simulink model "rocket_thrust_data_test"  (R2014a)
settings: Solver=ode45  StartTime=0.0  StopTime=1.3  MinStep=0.01  RelTol=1e-3
libraries: rocket_thrust_data_library x1, rocket_dynamic_data_library x1
settings Model: Creator=scorpii  LastModifiedBy=scorpii
settings SolverCC: InitialStep=0.01

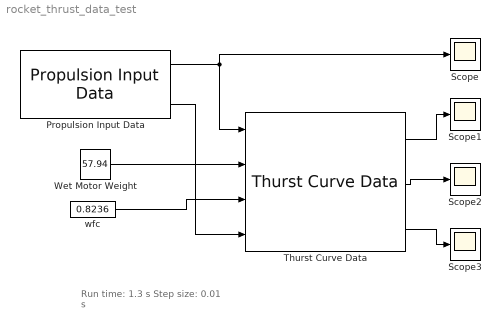
== system rocket_thrust_data_test ==
  note: Run time: 1.3 s
      | Step size: 0.01 s
  Propulsion Input Data : rocket_thrust_data_library/Propulsion Input Data
      link override Provided Specific Fuel Consumption: Value=0.0005387
  Scope{,1..3} (4 alike) : Scope
      Scope1 settings: YMin=0  YMax=2400
      Scope2 settings: YMin=48  YMax=58  SaveName=ScopeData2
      Scope3 settings: SaveName=ScopeData3
  Thurst Curve Data : rocket_dynamic_data_library/Thurst Curve Data
  Wet Motor Weight : Constant  Value=57.94
  wfc : Constant  Value=0.8236
  wires:
  Propulsion Input Data/1 -> Thurst Curve Data/1, Scope/1
  wfc/1 -> Thurst Curve Data/3
  Wet Motor Weight/1 -> Thurst Curve Data/2
  Thurst Curve Data/1 -> Scope1/1
  Thurst Curve Data/2 -> Scope2/1
  Thurst Curve Data/3 -> Scope3/1
  Propulsion Input Data/3 -> Thurst Curve Data/4
